simulink model "calcCylinderVolume"  (R2025b)
settings: Solver=VariableStepAuto  StartTime=0.0  StopTime=10.0  RelTol=1e-3
undefined symbols (not defined in the file): di, hi
settings Model: Creator=horiz  LastModifiedBy=horiz

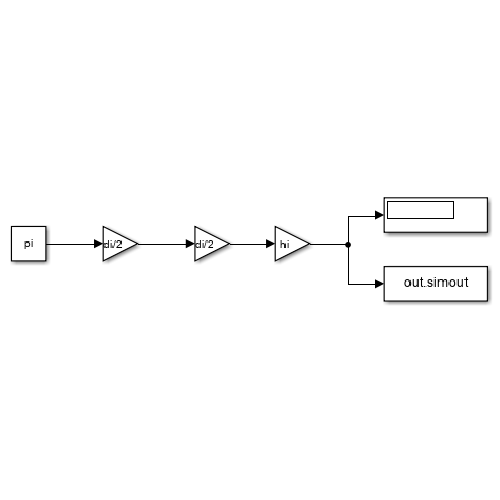
[thumbnail: Simulink's stored preview of the top-level diagram]
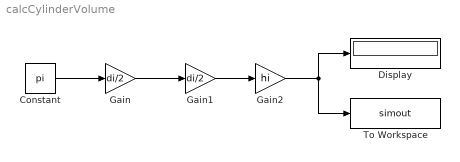
== system calcCylinderVolume ==
  Constant : Constant  Value=pi
  Display : Display
  Gain : Gain  Gain=di/2
  Gain1 : Gain  Gain=di/2
  Gain2 : Gain  Gain=hi
  To Workspace : ToWorkspace  VariableName=simout  SaveFormat=Timeseries  SampleTime=-1
  wires:
  Constant/1 -> Gain/1
  Gain/1 -> Gain1/1
  Gain1/1 -> Gain2/1
  Gain2/1 -> To Workspace/1, Display/1
